simulink model "ofdm"  (R2012b)
settings: Solver=FixedStepDiscrete  SolverMode=SingleTasking  StartTime=0.0  StopTime=500  RelTol=1e-3
undefined symbols (not defined in the file): a, addr, b, Down, Floor, Truncate, Up
libraries: shlslibv1 x120
settings Model: synDspstartup=OK  Creator=sszilvasi  LastModifiedBy=sszilvasi
settings DataIOCC: SaveOutput=off  SignalLogging=off  SaveTime=off
settings OptimizationCC: InlineParams=on
settings DebuggingCC: AlgebraicLoopMsg=error  InheritedTsInSrcMsg=none

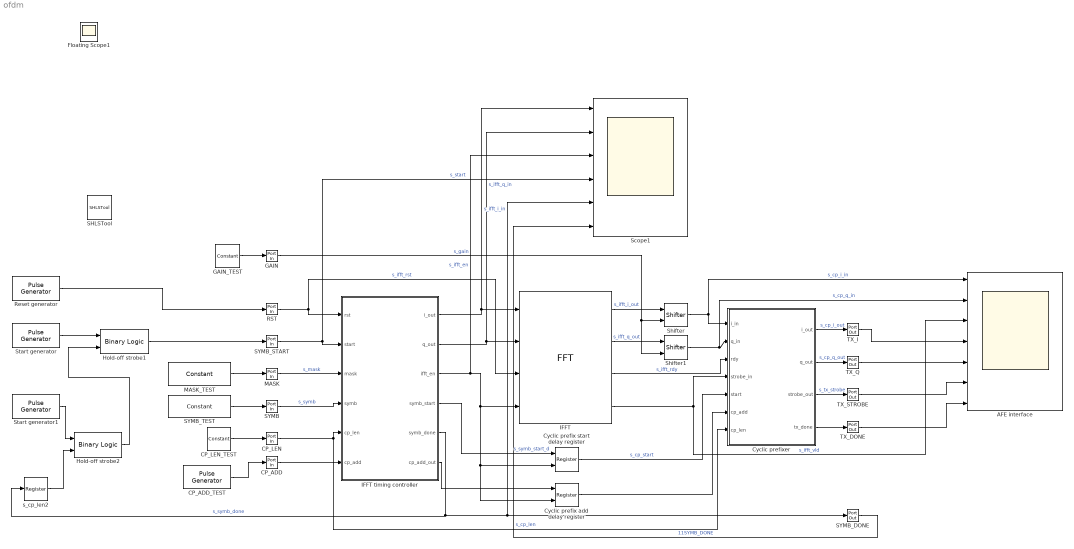
== system ofdm ==
  AFE interface : Scope  NumInputPorts=7
      settings: YMin=-0.04~-0.04~-1~-0.04~-0.04~-1~-1  YMax=0.04~0.04~2~0.04~0.04~2~2
  CP_ADD : shlslibv1/Ports & Subsystems/Port In  syn_out_wl=1  syn_out_fl=0  syn_out_dt=unsigned  syn_out_st=1  syn_capture=off  syn_register=off  syn_out_sat=off  syn_out_rnd=on  synBlockType=port  synLatency=0  synBlockId=0
  CP_ADD_TEST : shlslibv1/Sources/Pulse Generator  syn_siggentype=Step (0 to 1)  syn_usectl=off  syn_trigedge=rising  syn_triginit=low  syn_stpdel=120  syn_impwidth=1  syn_impdel=1  syn_st=1  synBlockType=custom  synLatency=0
  CP_LEN : shlslibv1/Ports & Subsystems/Port In  syn_out_wl=5  syn_out_fl=0  syn_out_dt=unsigned  syn_out_st=1  syn_capture=off  syn_register=off  syn_out_sat=off  syn_out_rnd=off  synBlockType=port  synLatency=0  synBlockId=0
  CP_LEN_TEST : shlslibv1/Sources/Constant  syn_cst_val=8  syn_cst_fl=0  syn_cst_dt=unsigned  syn_cst_rnd=off  syn_cst_st=-1  synBlockType=primitive  synLatency=0  synBlockId=15
  Cyclic prefix add delay register : shlslibv1/Memories/Register  syn_delay_val=71  syn_rst_port=off  syn_en_port=on  synBlockType=custom  synLatency=71
  Cyclic prefix start delay register : shlslibv1/Memories/Register  syn_delay_val=71  syn_rst_port=off  syn_en_port=on  synBlockType=custom  synLatency=71
  Cyclic prefixer : Subsystem
  GAIN : shlslibv1/Ports & Subsystems/Port In  syn_out_wl=2  syn_out_fl=0  syn_out_dt=unsigned  syn_out_st=1  syn_capture=off  syn_register=off  syn_out_sat=off  syn_out_rnd=on  synBlockType=port  synLatency=0  synBlockId=0
  GAIN_TEST : shlslibv1/Sources/Constant  syn_cst_val=0  syn_cst_fl=0  syn_cst_dt=unsigned  syn_cst_rnd=off  syn_cst_st=-1  synBlockType=primitive  synLatency=0  synBlockId=15
  Hold-off strobe1 : shlslibv1/Math Functions/Binary Logic  syn_binlog_exp=a|b  synBlockType=primitive  synLatency=0  synBlockId=13
  Hold-off strobe2 : shlslibv1/Math Functions/Binary Logic  syn_binlog_exp=a&b  synBlockType=primitive  synLatency=0  synBlockId=13
  IFFT : shlslibv1/Transforms/FFT  syn_fft_size=32  syn_fft_opr=Inverse  syn_real=on  syn_scale=Scale by 1/N  syn_twid_fl=10  syn_dp_f=Automatic  syn_dp_wl=syn_inp_wl  syn_dp_fl=syn_inp_fl  syn_dp_sat=off  syn_dp_round=Floor(Truncate)  syn_out_order=Natural  syn_out_f=Specify  syn_out_wl=13  syn_out_fl=12  syn_out_dt=signed  syn_out_sat=off  syn_out_round=Floor(Truncate)  syn_rst_port=on  syn_en_port=on  syn_rdy_port=on  syn_vld_port=on  synBlockType=primitive  synLatency=71  synBlockId=77
  IFFT timing controller : Subsystem
  MASK : shlslibv1/Ports & Subsystems/Port In  syn_out_wl=32  syn_out_fl=0  syn_out_dt=unsigned  syn_out_st=1  syn_capture=off  syn_register=off  syn_out_sat=off  syn_out_rnd=off  synBlockType=port  synLatency=0  synBlockId=0
  MASK_TEST : shlslibv1/Sources/Constant  syn_cst_val=hex2dec('00004000')  syn_cst_fl=0  syn_cst_dt=unsigned  syn_cst_rnd=off  syn_cst_st=-1  synBlockType=primitive  synLatency=0  synBlockId=15
  RST : shlslibv1/Ports & Subsystems/Port In  syn_out_wl=1  syn_out_fl=0  syn_out_dt=unsigned  syn_out_st=1  syn_capture=off  syn_register=off  syn_out_sat=off  syn_out_rnd=on  synBlockType=port  synLatency=0  synBlockId=0
  Reset generator : shlslibv1/Sources/Pulse Generator  syn_siggentype=Impulse  syn_usectl=off  syn_trigedge=rising  syn_triginit=low  syn_stpdel=10  syn_impwidth=1  syn_impdel=1  syn_st=1  synBlockType=custom  synLatency=0
  SHLSTool : shlslibv1/SHLSTool  synBlockType=tool  syn_dsp_mode=FPGA
  SYMB : shlslibv1/Ports & Subsystems/Port In  syn_out_wl=32  syn_out_fl=0  syn_out_dt=unsigned  syn_out_st=1  syn_capture=off  syn_register=off  syn_out_sat=off  syn_out_rnd=off  synBlockType=port  synLatency=0  synBlockId=0
  SYMB_DONE : shlslibv1/Ports & Subsystems/Port Out  syn_capture=off  syn_register=on  synBlockType=port  synLatency=1  synBlockId=1
  SYMB_START : shlslibv1/Ports & Subsystems/Port In  syn_out_wl=1  syn_out_fl=0  syn_out_dt=unsigned  syn_out_st=1  syn_capture=off  syn_register=off  syn_out_sat=off  syn_out_rnd=on  synBlockType=port  synLatency=0  synBlockId=0
  SYMB_TEST : shlslibv1/Sources/Constant  syn_cst_val=hex2dec('00008000')  syn_cst_fl=0  syn_cst_dt=unsigned  syn_cst_rnd=off  syn_cst_st=-1  synBlockType=primitive  synLatency=0  synBlockId=15
  Scope1 : Scope  NumInputPorts=6
      settings: YMin=-0.04~-0.04~-1~-0.04~-0.04~-1  YMax=0.04~0.04~2~0.04~0.04~2
  Shifter : shlslibv1/Math Functions/Shifter  syn_shifter_opr=<<  syn_out_f=Specify  syn_out_wl=10  syn_out_fl=9  syn_out_dt=signed  synBlockType=primitive  synLatency=0  synBlockId=12
  Shifter1 : shlslibv1/Math Functions/Shifter  syn_shifter_opr=<<  syn_out_f=Specify  syn_out_wl=10  syn_out_fl=9  syn_out_dt=signed  synBlockType=primitive  synLatency=0  synBlockId=12
  Start generator : shlslibv1/Sources/Pulse Generator  syn_siggentype=Impulse  syn_usectl=off  syn_trigedge=rising  syn_triginit=low  syn_stpdel=10  syn_impwidth=1  syn_impdel=2  syn_st=1  synBlockType=custom  synLatency=0
  Start generator1 : shlslibv1/Sources/Pulse Generator  syn_siggentype=Step (1 to 0)  syn_usectl=off  syn_trigedge=rising  syn_triginit=low  syn_stpdel=280  syn_impwidth=1  syn_impdel=200  syn_st=1  synBlockType=custom  synLatency=0
  TX_DONE : shlslibv1/Ports & Subsystems/Port Out  syn_capture=off  syn_register=on  synBlockType=port  synLatency=1  synBlockId=1
  TX_I : shlslibv1/Ports & Subsystems/Port Out  syn_capture=off  syn_register=on  synBlockType=port  synLatency=1  synBlockId=1
  TX_Q : shlslibv1/Ports & Subsystems/Port Out  syn_capture=off  syn_register=on  synBlockType=port  synLatency=1  synBlockId=1
  TX_STROBE : shlslibv1/Ports & Subsystems/Port Out  syn_capture=off  syn_register=on  synBlockType=port  synLatency=1  synBlockId=1
  s_cp_len2 : shlslibv1/Memories/Register  syn_delay_val=2  syn_rst_port=off  syn_en_port=off  synBlockType=custom  synLatency=2
  Floating Scope1 : Scope
      settings: Floating=on  SaveName=ScopeData10
  wires:
  RST/1 -> IFFT timing controller/1(rst), IFFT/3  "s_ifft_rst"
  IFFT/2 -> Shifter1/1  "s_ifft_q_out"
  IFFT/1 -> Shifter/1  "s_ifft_i_out"
  Cyclic prefixer/1(i_out) -> TX_I/1  "s_cp_i_out"
  Cyclic prefixer/2(q_out) -> TX_Q/1  "s_cp_q_out"
  IFFT/4 -> AFE interface/3, Cyclic prefixer/4(strobe_in)  "s_ifft_vld"
  IFFT/3 -> Cyclic prefixer/3(rdy)  "s_ifft_rdy"
  Cyclic prefix start delay register/1 -> Cyclic prefixer/5(start)  "s_cp_start"
  Start generator/1 -> Hold-off strobe1/1
  SYMB_TEST/1 -> SYMB/1
  MASK_TEST/1 -> MASK/1
  CP_LEN_TEST/1 -> CP_LEN/1
  Reset generator/1 -> RST/1
  Hold-off strobe1/1 -> SYMB_START/1
  s_cp_len2/1 -> Hold-off strobe2/2
  Hold-off strobe2/1 -> Hold-off strobe1/2
  Start generator1/1 -> Hold-off strobe2/1
  GAIN_TEST/1 -> GAIN/1
  Shifter/1 -> Cyclic prefixer/1(i_in), AFE interface/1  "s_cp_i_in"
  Shifter1/1 -> AFE interface/2, Cyclic prefixer/2(q_in)  "s_cp_q_in"
  GAIN/1 -> Shifter1/2, Shifter/2  "s_gain"
  IFFT timing controller/3(ifft_en) -> Scope1/3, IFFT/4, Cyclic prefix add delay register/2, Cyclic prefix start delay register/2  "s_ifft_en"
  SYMB_START/1 -> Scope1/4, IFFT timing controller/2(start)  "s_start"
  MASK/1 -> IFFT timing controller/3(mask)  "s_mask"
  SYMB/1 -> IFFT timing controller/4(symb)  "s_symb"
  CP_LEN/1 -> IFFT timing controller/5(cp_len), Cyclic prefixer/7(cp_len)  "s_cp_len"
  IFFT timing controller/1(i_out) -> Scope1/1, IFFT/1  "s_ifft_i_in"
  IFFT timing controller/2(q_out) -> Scope1/2, IFFT/2  "s_ifft_q_in"
  IFFT timing controller/4(symb_start) -> Cyclic prefix start delay register/1  "s_symb_start_d"
  IFFT timing controller/5(symb_done) -> Scope1/5, SYMB_DONE/1, s_cp_len2/1  "s_symb_done"
  Cyclic prefixer/3(strobe_out) -> TX_STROBE/1  "s_tx_strobe"
  TX_I/1 -> AFE interface/4
  TX_Q/1 -> AFE interface/5
  TX_STROBE/1 -> AFE interface/6
  IFFT timing controller/6(cp_add_out) -> Cyclic prefix add delay register/1
  Cyclic prefix add delay register/1 -> Cyclic prefixer/6(cp_add)
  CP_ADD/1 -> IFFT timing controller/6(cp_add)
  CP_ADD_TEST/1 -> CP_ADD/1
  Cyclic prefixer/4(tx_done) -> TX_DONE/1
  TX_DONE/1 -> AFE interface/7
  SYMB_DONE/1 -> Scope1/6  "11SYMB_DONE"

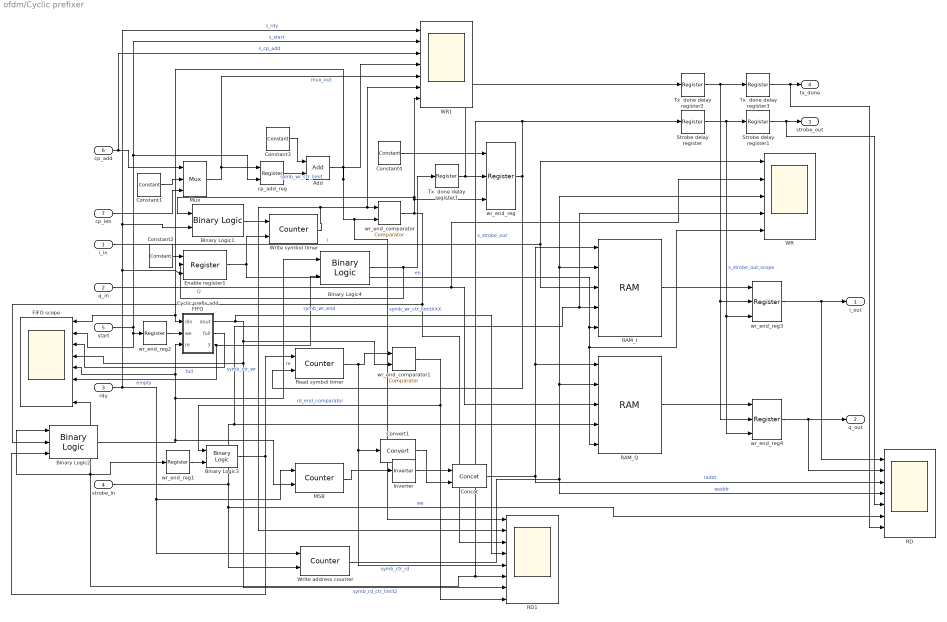
== system ofdm/Cyclic prefixer ==
  i_in : Inport
  q_in : Inport  Port=2
  rdy : Inport  Port=3
  strobe_in : Inport  Port=4
  start : Inport  Port=5
  cp_add : Inport  Port=6
  cp_len : Inport  Port=7
  Add : shlslibv1/Math Functions/Add  syn_add_opr=++  syn_out_f=Full Precision  syn_out_wl=16  syn_out_fl=8  syn_out_dt=signed  syn_out_sat=off  syn_out_rnd=Floor (Truncate)  synBlockType=primitive  synLatency=0  synBlockId=96  syn_sum_of_rows=off  syn_inh_port=off  syn_inh_st=off  syn_inh_stf=1
  Binary Logic1 : shlslibv1/Math Functions/Binary Logic  syn_binlog_exp=a | b  synBlockType=primitive  synLatency=0  synBlockId=13
  Binary Logic2 : shlslibv1/Math Functions/Binary Logic  syn_binlog_exp=(~a&b)|c  synBlockType=primitive  synLatency=0  synBlockId=13
  Binary Logic3 : shlslibv1/Math Functions/Binary Logic  syn_binlog_exp=a&b  synBlockType=primitive  synLatency=0  synBlockId=13
  Binary Logic4 : shlslibv1/Math Functions/Binary Logic  syn_binlog_exp=a&b  synBlockType=primitive  synLatency=0  synBlockId=13
  Concat : shlslibv1/Signal Operations/Concat  syn_in_nb=2  syn_out_f=Specify  syn_out_wl=6  syn_out_fl=0  syn_out_dt=unsigned  synBlockType=primitive  synLatency=0  synBlockId=8
  Constant1 : shlslibv1/Sources/Constant  syn_cst_val=0  syn_cst_fl=0  syn_cst_dt=unsigned  syn_cst_rnd=on  syn_cst_st=-1  synBlockType=primitive  synLatency=0  synBlockId=15
  Constant2 : shlslibv1/Sources/Constant  syn_cst_val=1  syn_cst_fl=0  syn_cst_dt=unsigned  syn_cst_rnd=on  syn_cst_st=-1  synBlockType=primitive  synLatency=0  synBlockId=15
  Constant3 : shlslibv1/Sources/Constant  syn_cst_val=32-1  syn_cst_fl=0  syn_cst_dt=unsigned  syn_cst_rnd=on  syn_cst_st=-1  synBlockType=primitive  synLatency=0  synBlockId=15
  Constant4 : shlslibv1/Sources/Constant  syn_cst_val=1  syn_cst_fl=0  syn_cst_dt=unsigned  syn_cst_rnd=on  syn_cst_st=-1  synBlockType=primitive  synLatency=0  synBlockId=15
  Convert1 : shlslibv1/Signal Operations/Convert  syn_preshift_opr=none  syn_preshift_bits=0  syn_preshift_val=0  syn_out_f=Specify  syn_out_wl=5  syn_out_fl=0  syn_out_dt_sync=unsigned  syn_out_sat=off  syn_out_rnd=Floor (Truncate)  syn_inh_port=off  syn_inh_st=off  syn_inh_stf=1  synBlockType=primitive  synLatency=0  synBlockId=4
  Cyclic prefix add FIFO : Subsystem
  Enable register1 : shlslibv1/Memories/Register  syn_delay_val=1  syn_rst_port=on  syn_en_port=on  synBlockType=custom  synLatency=1
  FIFO scope : Scope  NumInputPorts=8
      settings: YMin=-1~-1~-1~-1~-1~-1~-5~-5  YMax=41~2~2~41~2~2~5~5  SaveName=ScopeData6
  Inverter : shlslibv1/Math Functions/Inverter  syn_out_f=Automatic  syn_out_wl=16  syn_out_fl=8  syn_out_dt=signed  synBlockType=primitive  synLatency=0  synBlockId=10
  MSB : shlslibv1/Sources/Counter  syn_rst_port=on  syn_en_port=on  syn_ld_port=off  syn_cnt_type=Up  syn_init_val=0  syn_term_exists=off  syn_rdy_port=off  syn_term_val=127  syn_cnt_f=Specify  syn_cnt_wl=1  syn_cnt_dt=unsigned  syn_cnt_st=-1  synBlockType=primitive  synLatency=0  synBlockId=21
  Mux : shlslibv1/Signal Operations/Mux  syn_in_nb=2  syn_out_f=Full Precision  syn_out_wl=16  syn_out_fl=8  syn_out_dt=signed  synBlockType=primitive  synLatency=0  synBlockId=16
  RAM_I : shlslibv1/Memories/RAM  syn_ram_depth=64  syn_read_nb=1  syn_write_nb=1  syn_rw_nb=0  syn_corereset=off  syn_localreset=off  syn_initial_val=0  syn_enable_port=on  syn_wac=No check  syn_rac=Read-first  synBlockType=primitive  synLatency=1  synBlockId=111
  RAM_Q : shlslibv1/Memories/RAM  syn_ram_depth=64  syn_read_nb=1  syn_write_nb=1  syn_rw_nb=0  syn_corereset=off  syn_localreset=off  syn_initial_val=0  syn_enable_port=on  syn_wac=No check  syn_rac=Read-first  synBlockType=primitive  synLatency=1  synBlockId=111
  RD : Scope  NumInputPorts=7
      settings: YMin=-0.04~-0.04~0~-0~-1~-1~-5  YMax=0.04~0.04~65~65~2~2~5  SaveName=ScopeData4
  RD1 : Scope  NumInputPorts=8
      settings: YMin=-1~-1~-1~-1~-1~-1~-5~-5  YMax=41~41~2~41~41~2~5~5  SaveName=ScopeData5
  Read symbol timer : shlslibv1/Sources/Counter  syn_rst_port=on  syn_en_port=on  syn_ld_port=off  syn_cnt_type=Up  syn_init_val=0  syn_term_exists=off  syn_rdy_port=off  syn_term_val=127  syn_cnt_f=Specify  syn_cnt_wl=6  syn_cnt_dt=unsigned  syn_cnt_st=-1  synBlockType=primitive  synLatency=0  synBlockId=21
  Strobe delay register : shlslibv1/Memories/Register  syn_delay_val=1  syn_rst_port=off  syn_en_port=off  synBlockType=custom  synLatency=1
  Strobe delay register1 : shlslibv1/Memories/Register  syn_delay_val=1  syn_rst_port=off  syn_en_port=off  synBlockType=custom  synLatency=1
  Tx  done delay register1 : shlslibv1/Memories/Register  syn_delay_val=1  syn_rst_port=off  syn_en_port=off  synBlockType=custom  synLatency=1
  Tx  done delay register2 : shlslibv1/Memories/Register  syn_delay_val=1  syn_rst_port=off  syn_en_port=off  synBlockType=custom  synLatency=1
  Tx  done delay register3 : shlslibv1/Memories/Register  syn_delay_val=1  syn_rst_port=off  syn_en_port=off  synBlockType=custom  synLatency=1
  WR : Scope  NumInputPorts=5
      settings: YMin=-0.04~-0.04~0~-5~-5  YMax=0.04~0.04~5~5~5  SaveName=ScopeData3
  WR1 : Scope  NumInputPorts=7
      settings: YMin=-1~-1~-1~-1~-1~-1~-1  YMax=2~2~2~41~9~65~2  SaveName=ScopeData2
  Write address counter : shlslibv1/Sources/Counter  syn_rst_port=on  syn_en_port=on  syn_ld_port=off  syn_cnt_type=Up  syn_init_val=0  syn_term_exists=off  syn_rdy_port=off  syn_term_val=127  syn_cnt_f=Specify  syn_cnt_wl=6  syn_cnt_dt=unsigned  syn_cnt_st=-1  synBlockType=primitive  synLatency=0  synBlockId=21
  Write symbol timer : shlslibv1/Sources/Counter  syn_rst_port=on  syn_en_port=on  syn_ld_port=off  syn_cnt_type=Up  syn_init_val=0  syn_term_exists=off  syn_rdy_port=off  syn_term_val=127  syn_cnt_f=Specify  syn_cnt_wl=6  syn_cnt_dt=unsigned  syn_cnt_st=-1  synBlockType=primitive  synLatency=0  synBlockId=21
  cp_add_reg : shlslibv1/Memories/Register  syn_delay_val=1  syn_rst_port=off  syn_en_port=on  synBlockType=custom  synLatency=1
  wr_end_comparator : shlslibv1/Math Functions/Comparator  syn_comp_opr=a==b  syn_comp_const=off  syn_comp_val=2  synBlockType=primitive  synLatency=0  synBlockId=14
  wr_end_comparator1 : shlslibv1/Math Functions/Comparator  syn_comp_opr=a==b  syn_comp_const=off  syn_comp_val=2  synBlockType=primitive  synLatency=0  synBlockId=14
  wr_end_reg : shlslibv1/Memories/Register  syn_delay_val=1  syn_rst_port=on  syn_en_port=on  synBlockType=custom  synLatency=1
  wr_end_reg1 : shlslibv1/Memories/Register  syn_delay_val=1  syn_rst_port=off  syn_en_port=off  synBlockType=custom  synLatency=1
  wr_end_reg2 : shlslibv1/Memories/Register  syn_delay_val=1  syn_rst_port=off  syn_en_port=off  synBlockType=custom  synLatency=1
  wr_end_reg3 : shlslibv1/Memories/Register  syn_delay_val=1  syn_rst_port=on  syn_en_port=on  synBlockType=custom  synLatency=1
  wr_end_reg4 : shlslibv1/Memories/Register  syn_delay_val=1  syn_rst_port=on  syn_en_port=on  synBlockType=custom  synLatency=1
  i_out : Outport
  q_out : Outport  Port=2
  strobe_out : Outport  Port=3
  tx_done : Outport  Port=4
  wires:
  Write address counter/1 -> RAM_Q/2, WR/3, RAM_I/2, RD/4  "waddr"
  i_in/1 -> WR/1, RAM_I/3  "I"
  q_in/1 -> RAM_Q/3, WR/2  "Q"
  strobe_in/1 -> RD/6, Write address counter/2, WR/4, RAM_I/4, RAM_Q/4  "we"
  Convert1/1 -> Concat/2
  Concat/1 -> RAM_I/1, RAM_Q/1, RD/3  "raddr"
  MSB/1 -> Inverter/1
  rdy/1 -> Binary Logic1/2, WR1/1, Enable register1/3, Write address counter/1, MSB/1  "s_rdy"
  start/1 -> cp_add_reg/2, WR1/2, FIFO scope/2, wr_end_reg2/1  "s_start"
  cp_add/1 -> Mux/1, WR1/3  "s_cp_add"
  cp_len/1 -> Mux/3
  Constant1/1 -> Mux/2
  Mux/1 -> cp_add_reg/1, WR1/5  "mux_out"
  Constant2/1 -> Enable register1/1
  Write symbol timer/1 -> WR1/6, wr_end_comparator/1, RD1/2  "symb_ctr_wr"
  wr_end_comparator/1 -> WR1/7, Binary Logic1/1, wr_end_reg/3, Binary Logic2/2, RD1/3  "symb_wr_end"
  Constant3/1 -> Add/1
  Add/1 -> RD1/1, wr_end_comparator/2, Cyclic prefix add FIFO/1(din), FIFO scope/1, WR1/4  "symb_wr_ctr_limitXXX"
  Binary Logic1/1 -> Write symbol timer/1
  Constant4/1 -> wr_end_reg/1
  wr_end_reg/1 -> Read symbol timer/2, Strobe delay register/1, RD1/6, wr_end_reg1/1, Binary Logic2/1, FIFO scope/8  "s_strobe_out"
  cp_add_reg/1 -> Add/2  "symb_wr_ctr_limit"
  Cyclic prefix add FIFO/1(dout) -> RD1/4, wr_end_comparator1/2, FIFO scope/4, RD1/7  "symb_rd_ctr_limit2"
  Read symbol timer/1 -> wr_end_comparator1/1, Convert1/1, RD1/5  "symb_ctr_rd"
  Cyclic prefix add FIFO/2(full) -> FIFO scope/3  "full"
  Cyclic prefix add FIFO/3(empty) -> FIFO scope/6, Binary Logic4/2  "empty"
  Binary Logic2/1 -> MSB/2, Binary Logic4/1, Cyclic prefix add FIFO/3(re), FIFO scope/5  "re"
  wr_end_comparator1/1 -> Binary Logic3/1, RD1/8  "rd_end_comparator"
  wr_end_reg1/1 -> Binary Logic3/2
  Binary Logic3/1 -> Binary Logic2/3, Read symbol timer/1
  wr_end_reg2/1 -> Cyclic prefix add FIFO/2(we)
  Enable register1/1 -> RAM_I/5, WR/5, RAM_Q/5, Write symbol timer/2  "en"
  Inverter/1 -> Concat/1
  Strobe delay register/1 -> Strobe delay register1/1, wr_end_reg4/3, wr_end_reg3/3  "s_strobe_out_scope"
  Tx  done delay register1/1 -> wr_end_reg/2, Tx  done delay register2/1
  RAM_I/1 -> wr_end_reg3/1
  wr_end_reg3/1 -> i_out/1, RD/1
  wr_end_reg4/1 -> RD/2, q_out/1
  Binary Logic4/1 -> Enable register1/2, Tx  done delay register1/1
  Strobe delay register1/1 -> RD/5, strobe_out/1
  Tx  done delay register2/1 -> Tx  done delay register3/1, wr_end_reg4/2, wr_end_reg3/2
  RAM_Q/1 -> wr_end_reg4/1
  Tx  done delay register3/1 -> RD/7, tx_done/1

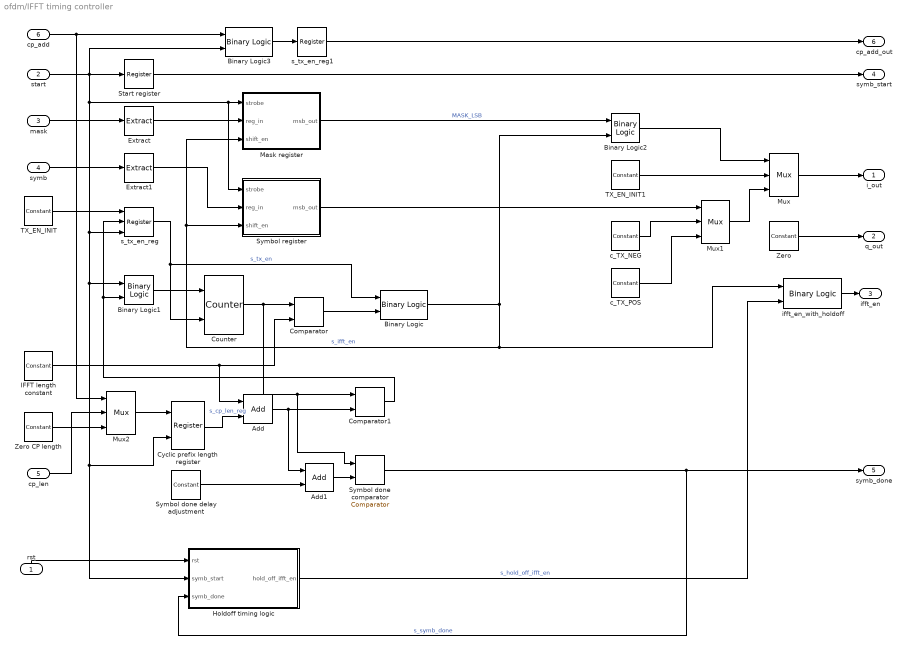
== system ofdm/IFFT timing controller ==
  rst : Inport
  start : Inport  Port=2
  mask : Inport  Port=3
  symb : Inport  Port=4
  cp_len : Inport  Port=5
  cp_add : Inport  Port=6
  Add : shlslibv1/Math Functions/Add  syn_add_opr=++  syn_out_f=Full Precision  syn_out_wl=16  syn_out_fl=8  syn_out_dt=signed  syn_out_sat=off  syn_out_rnd=Floor (Truncate)  synBlockType=primitive  synLatency=0  synBlockId=96  syn_sum_of_rows=off  syn_inh_port=off  syn_inh_st=off  syn_inh_stf=1
  Add1 : shlslibv1/Math Functions/Add  syn_add_opr=+-  syn_out_f=Full Precision  syn_out_wl=16  syn_out_fl=8  syn_out_dt=signed  syn_out_sat=off  syn_out_rnd=Floor (Truncate)  synBlockType=primitive  synLatency=0  synBlockId=96  syn_sum_of_rows=off  syn_inh_port=off  syn_inh_st=off  syn_inh_stf=1
  Binary Logic : shlslibv1/Math Functions/Binary Logic  syn_binlog_exp=a&b  synBlockType=primitive  synLatency=0  synBlockId=13
  Binary Logic1 : shlslibv1/Math Functions/Binary Logic  syn_binlog_exp=a|b  synBlockType=primitive  synLatency=0  synBlockId=13
  Binary Logic2 : shlslibv1/Math Functions/Binary Logic  syn_binlog_exp=a&b  synBlockType=primitive  synLatency=0  synBlockId=13
  Binary Logic3 : shlslibv1/Math Functions/Binary Logic  syn_binlog_exp=a&b  synBlockType=primitive  synLatency=0  synBlockId=13
  Comparator : shlslibv1/Math Functions/Comparator  syn_comp_opr=a<b  syn_comp_const=off  syn_comp_val=31  synBlockType=primitive  synLatency=0  synBlockId=14
  Comparator1 : shlslibv1/Math Functions/Comparator  syn_comp_opr=a>=b  syn_comp_const=off  syn_comp_val=31  synBlockType=primitive  synLatency=0  synBlockId=14
  Counter : shlslibv1/Sources/Counter  syn_rst_port=on  syn_en_port=on  syn_ld_port=off  syn_cnt_type=Up  syn_init_val=0  syn_term_exists=off  syn_rdy_port=off  syn_term_val=127  syn_cnt_f=Specify  syn_cnt_wl=6  syn_cnt_dt=unsigned  syn_cnt_st=-1  synBlockType=primitive  synLatency=0  synBlockId=21
  Cyclic prefix length register : shlslibv1/Memories/Register  syn_delay_val=1  syn_rst_port=off  syn_en_port=on  synBlockType=custom  synLatency=1
  Extract : shlslibv1/Signal Operations/Extract  syn_extract_vec=[16:31 0:15]  synBlockType=primitive  synLatency=0  synBlockId=17
  Extract1 : shlslibv1/Signal Operations/Extract  syn_extract_vec=[16:31 0:15]  synBlockType=primitive  synLatency=0  synBlockId=17
  Holdoff timing logic : Subsystem
  IFFT length constant : shlslibv1/Sources/Constant  syn_cst_val=32  syn_cst_fl=0  syn_cst_dt=unsigned  syn_cst_rnd=off  syn_cst_st=-1  synBlockType=primitive  synLatency=0  synBlockId=15
  Mask register : Subsystem
  Mux : shlslibv1/Signal Operations/Mux  syn_in_nb=2  syn_out_f=Full Precision  syn_out_wl=16  syn_out_fl=8  syn_out_dt=signed  synBlockType=primitive  synLatency=0  synBlockId=16
  Mux1 : shlslibv1/Signal Operations/Mux  syn_in_nb=2  syn_out_f=Full Precision  syn_out_wl=16  syn_out_fl=8  syn_out_dt=signed  synBlockType=primitive  synLatency=0  synBlockId=16
  Mux2 : shlslibv1/Signal Operations/Mux  syn_in_nb=2  syn_out_f=Full Precision  syn_out_wl=16  syn_out_fl=8  syn_out_dt=signed  synBlockType=primitive  synLatency=0  synBlockId=16
  Start register : shlslibv1/Memories/Register  syn_delay_val=1  syn_rst_port=off  syn_en_port=off  synBlockType=custom  synLatency=1
  Symbol done comparator : shlslibv1/Math Functions/Comparator  syn_comp_opr=a==b  syn_comp_const=off  syn_comp_val=31  synBlockType=primitive  synLatency=0  synBlockId=14
  Symbol done delay adjustment : shlslibv1/Sources/Constant  syn_cst_val=3  syn_cst_fl=0  syn_cst_dt=unsigned  syn_cst_rnd=off  syn_cst_st=-1  synBlockType=primitive  synLatency=0  synBlockId=15
  Symbol register : Subsystem
  TX_EN_INIT : shlslibv1/Sources/Constant  syn_cst_val=1  syn_cst_fl=0  syn_cst_dt=unsigned  syn_cst_rnd=off  syn_cst_st=-1  synBlockType=primitive  synLatency=0  synBlockId=15
  TX_EN_INIT1 : shlslibv1/Sources/Constant  syn_cst_val=0  syn_cst_fl=3  syn_cst_dt=unsigned  syn_cst_rnd=off  syn_cst_st=-1  synBlockType=primitive  synLatency=0  synBlockId=15
  Zero : shlslibv1/Sources/Constant  syn_cst_val=0  syn_cst_fl=3  syn_cst_dt=signed  syn_cst_rnd=off  syn_cst_st=-1  synBlockType=primitive  synLatency=0  synBlockId=15
  Zero CP length : shlslibv1/Sources/Constant  syn_cst_val=0  syn_cst_fl=0  syn_cst_dt=unsigned  syn_cst_rnd=off  syn_cst_st=-1  synBlockType=primitive  synLatency=0  synBlockId=15
  c_TX_NEG : shlslibv1/Sources/Constant  syn_cst_val=-0.75  syn_cst_fl=3  syn_cst_dt=signed  syn_cst_rnd=off  syn_cst_st=-1  synBlockType=primitive  synLatency=0  synBlockId=15
  c_TX_POS : shlslibv1/Sources/Constant  syn_cst_val=0.75  syn_cst_fl=3  syn_cst_dt=signed  syn_cst_rnd=off  syn_cst_st=-1  synBlockType=primitive  synLatency=0  synBlockId=15
  ifft_en_with_holdoff : shlslibv1/Math Functions/Binary Logic  syn_binlog_exp=a|b  synBlockType=primitive  synLatency=0  synBlockId=13
  s_tx_en_reg : shlslibv1/Memories/Register  syn_delay_val=1  syn_rst_port=on  syn_en_port=on  synBlockType=custom  synLatency=1
  s_tx_en_reg1 : shlslibv1/Memories/Register  syn_delay_val=1  syn_rst_port=off  syn_en_port=off  synBlockType=custom  synLatency=1
  i_out : Outport
  q_out : Outport  Port=2
  ifft_en : Outport  Port=3
  symb_start : Outport  Port=4
  symb_done : Outport  Port=5
  cp_add_out : Outport  Port=6
  wires:
  mask/1 -> Extract/1
  Cyclic prefix length register/1 -> Add/2  "s_cp_len_reg"
  Symbol done delay adjustment/1 -> Add1/2
  c_TX_POS/1 -> Mux1/3
  Zero/1 -> q_out/1
  ifft_en_with_holdoff/1 -> ifft_en/1
  Add/1 -> Comparator1/2, Add1/1
  IFFT length constant/1 -> Comparator/2, Add/1
  Symbol done comparator/1 -> symb_done/1, Holdoff timing logic/3(symb_done)  "s_symb_done"
  Start register/1 -> symb_start/1
  Symbol register/1(msb_out) -> Mux1/1
  Binary Logic/1 -> Mask register/3(shift_en), Symbol register/3(shift_en), ifft_en_with_holdoff/1, Binary Logic2/2  "s_ifft_en"
  Extract/1 -> Mask register/2(reg_in)
  start/1 -> Binary Logic3/2, Symbol register/1(strobe), Mask register/1(strobe), Binary Logic1/1, Holdoff timing logic/2(symb_start), Cyclic prefix length register/2, s_tx_en_reg/3, Start register/1
  Counter/1 -> Comparator1/1, Symbol done comparator/1, Comparator/1
  Comparator1/1 -> Binary Logic1/2, s_tx_en_reg/2
  Binary Logic2/1 -> Mux/1
  Mux1/1 -> Mux/3
  TX_EN_INIT1/1 -> Mux/2
  TX_EN_INIT/1 -> s_tx_en_reg/1
  Holdoff timing logic/1(hold_off_ifft_en) -> ifft_en_with_holdoff/2  "s_hold_off_ifft_en"
  Add1/1 -> Symbol done comparator/2
  Mask register/1(msb_out) -> Binary Logic2/1  "MASK_LSB"
  Mux/1 -> i_out/1
  c_TX_NEG/1 -> Mux1/2
  Binary Logic1/1 -> Counter/1
  Extract1/1 -> Symbol register/2(reg_in)
  symb/1 -> Extract1/1
  s_tx_en_reg/1 -> Binary Logic/1, Counter/2  "s_tx_en"
  rst/1 -> Holdoff timing logic/1(rst)
  s_tx_en_reg1/1 -> cp_add_out/1
  cp_add/1 -> Mux2/1, Binary Logic3/1
  Binary Logic3/1 -> s_tx_en_reg1/1
  Comparator/1 -> Binary Logic/2
  Zero CP length/1 -> Mux2/2
  cp_len/1 -> Mux2/3
  Mux2/1 -> Cyclic prefix length register/1

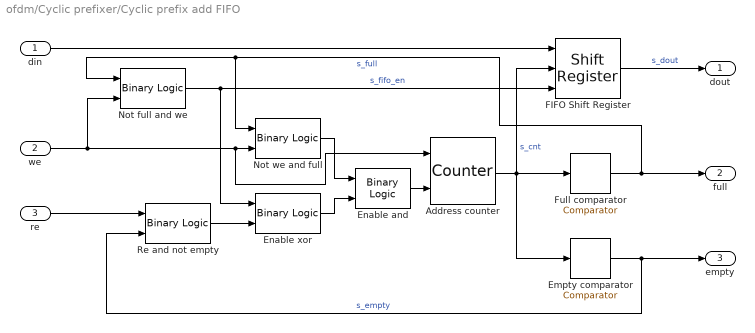
== system ofdm/Cyclic prefixer/Cyclic prefix add FIFO ==
  din : Inport
  we : Inport  Port=2
  re : Inport  Port=3
  Address counter : shlslibv1/Sources/Counter  syn_rst_port=off  syn_en_port=on  syn_ld_port=off  syn_cnt_type=Up/Down  syn_init_val=0  syn_term_exists=off  syn_rdy_port=off  syn_term_val=127  syn_cnt_f=Specify  syn_cnt_wl=2  syn_cnt_dt=unsigned  syn_cnt_st=1  synBlockType=primitive  synLatency=0  synBlockId=21
  Empty comparator : shlslibv1/Math Functions/Comparator  syn_comp_opr=a==b  syn_comp_const=on  syn_comp_val=0  synBlockType=primitive  synLatency=0  synBlockId=14
  Enable and : shlslibv1/Math Functions/Binary Logic  syn_binlog_exp=a&b  synBlockType=primitive  synLatency=0  synBlockId=13
  Enable xor : shlslibv1/Math Functions/Binary Logic  syn_binlog_exp=a^b  synBlockType=primitive  synLatency=0  synBlockId=13
  FIFO Shift Register : shlslibv1/Memories/Shift Register  syn_shift_dynamic=on  syn_shift_vec=15  syn_shift_val=3  syn_vect_out=Normal  syn_rst_val=All zeros  syn_rst_vec=0  syn_rst_port=off  syn_en_port=on  synBlockType=primitive  synLatency=(addr+1)  synBlockId=93  syn_inp_passthrough=off
  Full comparator : shlslibv1/Math Functions/Comparator  syn_comp_opr=a==b  syn_comp_const=on  syn_comp_val=2  synBlockType=primitive  synLatency=0  synBlockId=14
  Not full and we : shlslibv1/Math Functions/Binary Logic  syn_binlog_exp=~a&b  synBlockType=primitive  synLatency=0  synBlockId=13
  Not we and full : shlslibv1/Math Functions/Binary Logic  syn_binlog_exp=~(a&b)  synBlockType=primitive  synLatency=0  synBlockId=13
  Re and not empty : shlslibv1/Math Functions/Binary Logic  syn_binlog_exp=a&~b  synBlockType=primitive  synLatency=0  synBlockId=13
  dout : Outport
  full : Outport  Port=2
  empty : Outport  Port=3
  wires:
  FIFO Shift Register/1 -> dout/1  "s_dout"
  we/1 -> Not full and we/2, Address counter/1, Not we and full/2
  Re and not empty/1 -> Enable xor/2
  Enable xor/1 -> Enable and/2
  din/1 -> FIFO Shift Register/1
  re/1 -> Re and not empty/1
  Address counter/1 -> FIFO Shift Register/2, Empty comparator/1, Full comparator/1  "s_cnt"
  Full comparator/1 -> full/1, Not we and full/1, Not full and we/1  "s_full"
  Not we and full/1 -> Enable and/1
  Enable and/1 -> Address counter/2
  Empty comparator/1 -> empty/1, Re and not empty/2  "s_empty"
  Not full and we/1 -> Enable xor/1, FIFO Shift Register/3  "s_fifo_en"

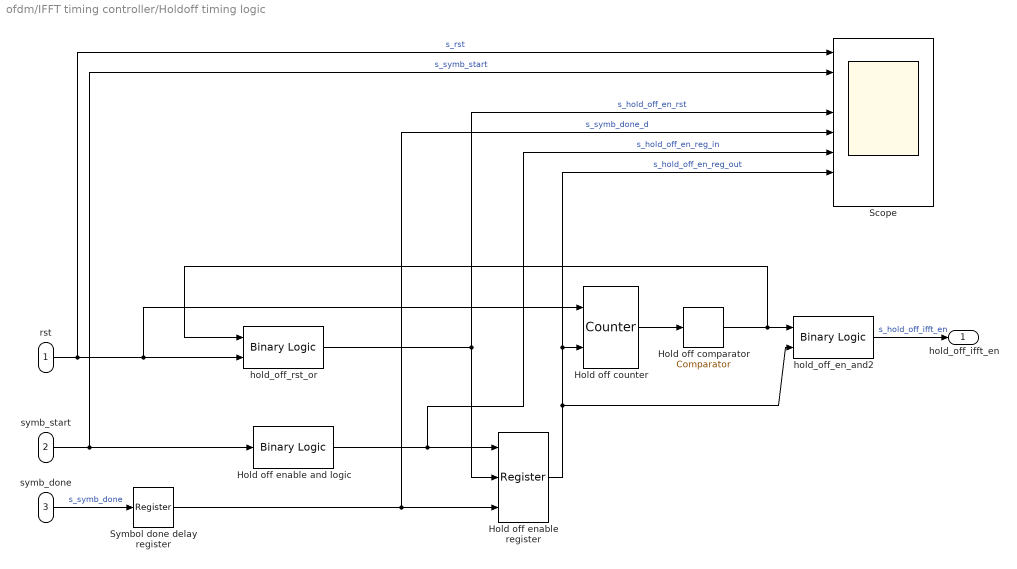
== system ofdm/IFFT timing controller/Holdoff timing logic ==
  rst : Inport
  symb_start : Inport  Port=2
  symb_done : Inport  Port=3
  Hold off comparator : shlslibv1/Math Functions/Comparator  syn_comp_opr=a>=b  syn_comp_const=on  syn_comp_val=71  synBlockType=primitive  synLatency=0  synBlockId=14
  Hold off counter : shlslibv1/Sources/Counter  syn_rst_port=on  syn_en_port=on  syn_ld_port=off  syn_cnt_type=Up  syn_init_val=0  syn_term_exists=off  syn_rdy_port=off  syn_term_val=15  syn_cnt_f=Specify  syn_cnt_wl=7  syn_cnt_dt=unsigned  syn_cnt_st=-1  synBlockType=primitive  synLatency=0  synBlockId=21
  Hold off enable register : shlslibv1/Memories/Register  syn_delay_val=1  syn_rst_port=on  syn_en_port=on  synBlockType=custom  synLatency=1
  Hold off enable and logic : shlslibv1/Math Functions/Binary Logic  syn_binlog_exp=~a  synBlockType=primitive  synLatency=0  synBlockId=13
  Scope : Scope  NumInputPorts=8
      settings: YMin=-5~-5~-5~-5~-5~-5~-5~-5  YMax=5~5~5~5~5~5~5~5  SaveName=ScopeData7
  Symbol done delay register : shlslibv1/Memories/Register  syn_delay_val=2  syn_rst_port=off  syn_en_port=off  synBlockType=custom  synLatency=2
  hold_off_en_and2 : shlslibv1/Math Functions/Binary Logic  syn_binlog_exp=~a&b  synBlockType=primitive  synLatency=0  synBlockId=13
  hold_off_rst_or : shlslibv1/Math Functions/Binary Logic  syn_binlog_exp=a|b  synBlockType=primitive  synLatency=0  synBlockId=13
  hold_off_ifft_en : Outport
  wires:
  symb_done/1 -> Symbol done delay register/1  "s_symb_done"
  symb_start/1 -> Scope/2, Hold off enable and logic/1  "s_symb_start"
  rst/1 -> Scope/1, hold_off_rst_or/2, Hold off counter/1  "s_rst"
  Hold off counter/1 -> Hold off comparator/1
  Hold off enable register/1 -> Hold off counter/2, Scope/7, hold_off_en_and2/2  "s_hold_off_en_reg_out"
  Hold off enable and logic/1 -> Scope/6, Hold off enable register/1  "s_hold_off_en_reg_in"
  hold_off_en_and2/1 -> hold_off_ifft_en/1  "s_hold_off_ifft_en"
  hold_off_rst_or/1 -> Hold off enable register/2, Scope/4  "s_hold_off_en_rst"
  Symbol done delay register/1 -> Scope/5, Hold off enable register/3  "s_symb_done_d"
  Hold off comparator/1 -> hold_off_rst_or/1, hold_off_en_and2/1

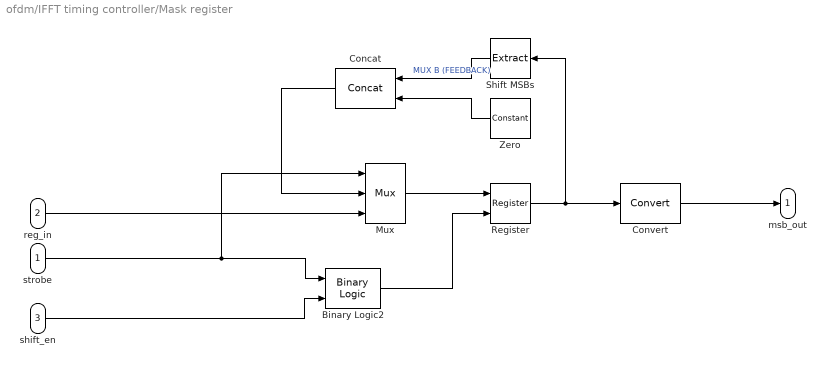
== system ofdm/IFFT timing controller/Mask register ==
  strobe : Inport
  reg_in : Inport  Port=2
  shift_en : Inport  Port=3
  Binary Logic2 : shlslibv1/Math Functions/Binary Logic  syn_binlog_exp=a|b  synBlockType=primitive  synLatency=0  synBlockId=13
  Concat : shlslibv1/Signal Operations/Concat  syn_in_nb=2  syn_out_f=Automatic  syn_out_wl=16  syn_out_fl=8  syn_out_dt=signed  synBlockType=primitive  synLatency=0  synBlockId=8
  Convert : shlslibv1/Signal Operations/Convert  syn_preshift_opr=>>  syn_preshift_bits=31  syn_preshift_val=0  syn_out_f=Specify  syn_out_wl=1  syn_out_fl=0  syn_out_dt_sync=unsigned  syn_out_sat=off  syn_out_rnd=Floor (Truncate)  syn_inh_port=off  syn_inh_st=off  syn_inh_stf=1  synBlockType=primitive  synLatency=0  synBlockId=4
  Mux : shlslibv1/Signal Operations/Mux  syn_in_nb=2  syn_out_f=Full Precision  syn_out_wl=16  syn_out_fl=8  syn_out_dt=signed  synBlockType=primitive  synLatency=0  synBlockId=16
  Register : shlslibv1/Memories/Register  syn_delay_val=1  syn_rst_port=off  syn_en_port=on  synBlockType=custom  synLatency=1
  Shift MSBs : shlslibv1/Signal Operations/Extract  syn_extract_vec=[0:30]  synBlockType=primitive  synLatency=0  synBlockId=17
  Zero : shlslibv1/Sources/Constant  syn_cst_val=0  syn_cst_fl=0  syn_cst_dt=unsigned  syn_cst_rnd=off  syn_cst_st=-1  synBlockType=primitive  synLatency=0  synBlockId=15
  msb_out : Outport
  wires:
  Convert/1 -> msb_out/1
  strobe/1 -> Mux/1, Binary Logic2/1
  shift_en/1 -> Binary Logic2/2
  reg_in/1 -> Mux/3
  Mux/1 -> Register/1
  Concat/1 -> Mux/2
  Binary Logic2/1 -> Register/2
  Register/1 -> Shift MSBs/1, Convert/1
  Zero/1 -> Concat/2
  Shift MSBs/1 -> Concat/1  "MUX B (FEEDBACK)"

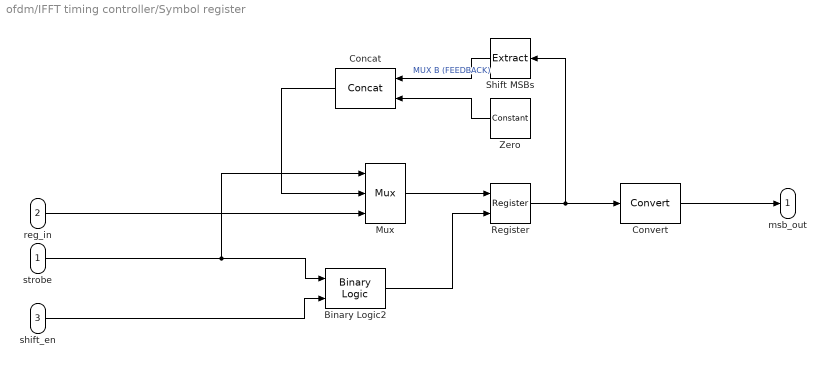
== system ofdm/IFFT timing controller/Symbol register ==
  strobe : Inport
  reg_in : Inport  Port=2
  shift_en : Inport  Port=3
  Binary Logic2 : shlslibv1/Math Functions/Binary Logic  syn_binlog_exp=a|b  synBlockType=primitive  synLatency=0  synBlockId=13
  Concat : shlslibv1/Signal Operations/Concat  syn_in_nb=2  syn_out_f=Automatic  syn_out_wl=16  syn_out_fl=8  syn_out_dt=signed  synBlockType=primitive  synLatency=0  synBlockId=8
  Convert : shlslibv1/Signal Operations/Convert  syn_preshift_opr=>>  syn_preshift_bits=31  syn_preshift_val=0  syn_out_f=Specify  syn_out_wl=1  syn_out_fl=0  syn_out_dt_sync=unsigned  syn_out_sat=off  syn_out_rnd=Floor (Truncate)  syn_inh_port=off  syn_inh_st=off  syn_inh_stf=1  synBlockType=primitive  synLatency=0  synBlockId=4
  Mux : shlslibv1/Signal Operations/Mux  syn_in_nb=2  syn_out_f=Full Precision  syn_out_wl=16  syn_out_fl=8  syn_out_dt=signed  synBlockType=primitive  synLatency=0  synBlockId=16
  Register : shlslibv1/Memories/Register  syn_delay_val=1  syn_rst_port=off  syn_en_port=on  synBlockType=custom  synLatency=1
  Shift MSBs : shlslibv1/Signal Operations/Extract  syn_extract_vec=[0:30]  synBlockType=primitive  synLatency=0  synBlockId=17
  Zero : shlslibv1/Sources/Constant  syn_cst_val=0  syn_cst_fl=0  syn_cst_dt=unsigned  syn_cst_rnd=off  syn_cst_st=-1  synBlockType=primitive  synLatency=0  synBlockId=15
  msb_out : Outport
  wires:
  Shift MSBs/1 -> Concat/1  "MUX B (FEEDBACK)"
  Zero/1 -> Concat/2
  Register/1 -> Convert/1, Shift MSBs/1
  Binary Logic2/1 -> Register/2
  Concat/1 -> Mux/2
  Mux/1 -> Register/1
  reg_in/1 -> Mux/3
  shift_en/1 -> Binary Logic2/2
  strobe/1 -> Binary Logic2/1, Mux/1
  Convert/1 -> msb_out/1
